simulink model "hw3q7"  (R2022b)
settings: Solver=ode1  StartTime=0.0  StopTime=10  FixedStep=0.01  RelTol=1e-3
settings Model: Creator=A  LastModifiedBy=asus
settings DebuggingCC: UnconnectedInputMsg=warning  UnconnectedOutputMsg=warning  UnconnectedLineMsg=warning
settings ModelReferenceCC: EnableRefExpFcnMdlSchedulingChecks=on
settings RTWCC: DLArmComputeVersion=19.05

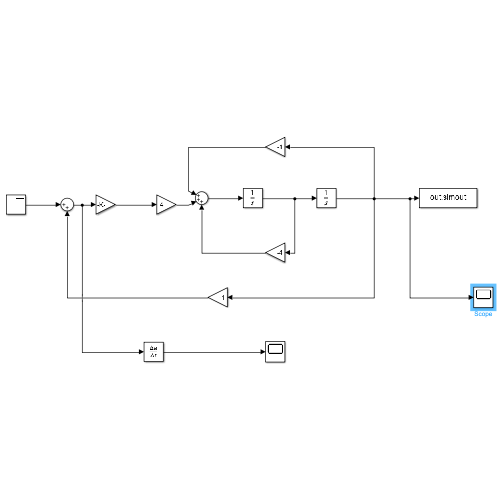
[thumbnail: Simulink's stored preview of the top-level diagram]
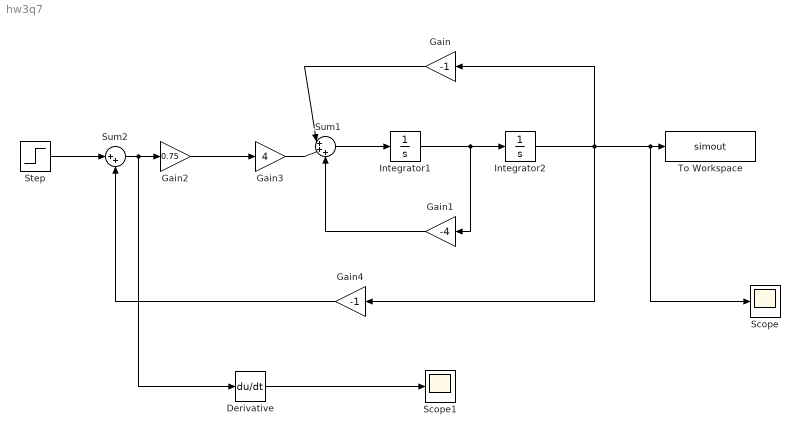
== system hw3q7 ==
  Derivative : Derivative
  Gain : Gain  Gain=-1
  Gain1 : Gain  Gain=-4
  Gain2 : Gain  Gain=0.75
  Gain3 : Gain  Gain=4
  Gain4 : Gain  Gain=-1
  Integrator1 : Integrator
  Integrator2 : Integrator
  Scope : Scope
  Scope1 : Scope
  Step : Step  Time=0  SampleTime=0
  Sum1 : Sum  Inputs=|+++
  Sum2 : Sum  Inputs=|++
  To Workspace : ToWorkspace  VariableName=simout  SaveFormat=Timeseries  SampleTime=-1
  wires:
  Sum1/1 -> Integrator1/1
  Sum2/1 -> Derivative/1, Gain2/1
  Step/1 -> Sum2/1
  Gain4/1 -> Sum2/2
  Gain2/1 -> Gain3/1
  Gain/1 -> Sum1/1
  Gain3/1 -> Sum1/2
  Gain1/1 -> Sum1/3
  Integrator1/1 -> Gain1/1, Integrator2/1
  Integrator2/1 -> Gain4/1, Scope/1, To Workspace/1, Gain/1
  Derivative/1 -> Scope1/1
